simulink model "gps_navsatfix_sim"  (R2026a)
settings: Solver=FixedStepDiscrete  StopTime=Inf  FixedStep=0.1
model workspace (MAT data in the model file):
  GPS_FIX_TOPIC = '/gps/fix'
  GPS_REFERENCE_LLA = [42.3 -71.35 20]
  GPS_SAMPLE_TIME = 0.1
  ODOM_TOPIC = '/odom'
undefined symbols (not defined in the file): altitude, latitude, longitude, position_covariance, position_covariance_type, status
libraries: sensorgpslib x4, ros2lib x4
settings Model: Creator=abshanka  LastModifiedBy=abshanka
settings HardwareCC: ProdBitPerLong=64.0  ProdHWDeviceType=Intel->x86-64 (Linux 64)
settings RTWCC: SystemTargetFile=ert.tlc  HardwareBoard=Robot Operating System 2 (ROS 2)  TLCOptions="-aInlineSetEventsForThisBaseRateFcn=TLC_FALSE -aSuppressMultiTaskScheduler=TLC_FALSE  -aRateBasedStepFcn=0"  Toolchain=Colcon Tools  TargetLang=C++  Description=Embedded Coder
settings ERTTargetCC: ExtModeTransport=2.0  ExtModeAutomaticAllocSize=off  RootIOFormat=Structure reference  CodeInterfacePackaging=C++ class

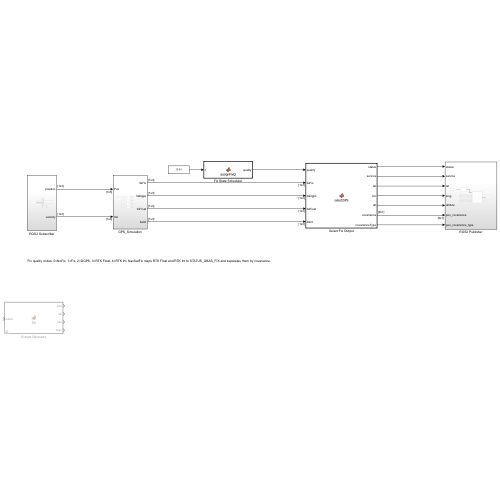
[thumbnail: Simulink's stored preview of the top-level diagram]
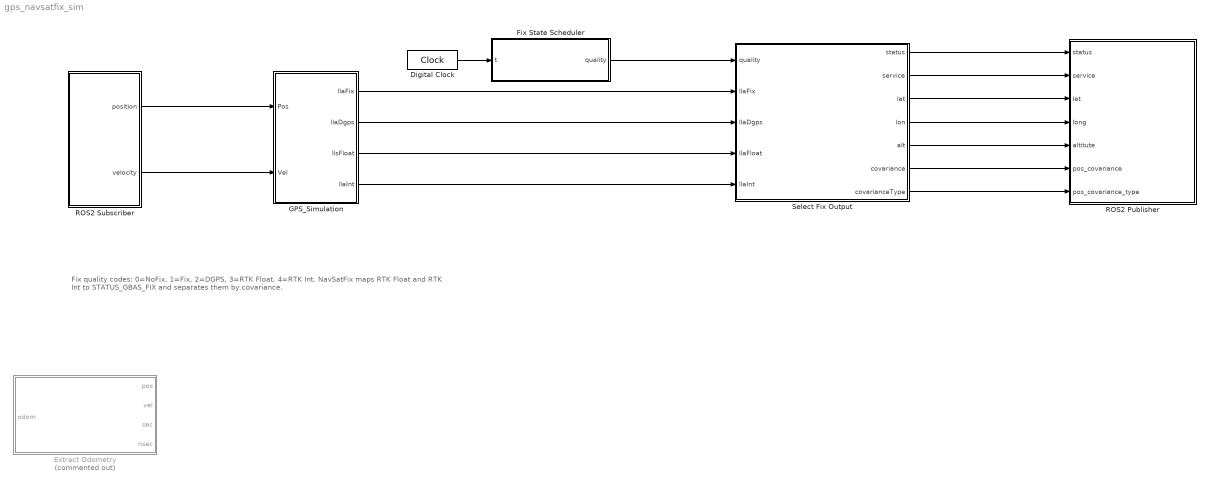
== system gps_navsatfix_sim ==
  note: Fix quality codes: 0=NoFix, 1=Fix, 2=DGPS, 3=RTK Float, 4=RTK Int. NavSatFix maps RTK Float and RTK Int to STATUS_GBAS_FIX and separates them by covariance.
  Digital Clock : DigitalClock  SampleTime=GPS_SAMPLE_TIME
  Extract Odometry : MATLAB Function  Commented=on  TreatAsAtomicUnit=on
  Fix State Scheduler : MATLAB Function  TreatAsAtomicUnit=on
  GPS_Simulation : Subsystem
  ROS2 Publisher : Subsystem
  ROS2 Subscriber : Subsystem
  Select Fix Output : MATLAB Function  TreatAsAtomicUnit=on
  wires:
  Digital Clock/1 -> Fix State Scheduler/1(t)
  Fix State Scheduler/1(quality) -> Select Fix Output/1(quality)
  GPS_Simulation/1(llaFix) -> Select Fix Output/2(llaFix)
  GPS_Simulation/2(llaDgps) -> Select Fix Output/3(llaDgps)
  GPS_Simulation/3(llsFloat) -> Select Fix Output/4(llaFloat)
  GPS_Simulation/4(llaInt) -> Select Fix Output/5(llaInt)
  ROS2 Subscriber/1(position) -> GPS_Simulation/1(Pos)
  ROS2 Subscriber/2(velocity) -> GPS_Simulation/2(Vel)
  Select Fix Output/1(status) -> ROS2 Publisher/1(status)
  Select Fix Output/2(service) -> ROS2 Publisher/2(service)
  Select Fix Output/3(lat) -> ROS2 Publisher/3(lat)
  Select Fix Output/4(lon) -> ROS2 Publisher/4(long)
  Select Fix Output/5(alt) -> ROS2 Publisher/5(altitute)
  Select Fix Output/6(covariance) -> ROS2 Publisher/6(pos_covariance)
  Select Fix Output/7(covarianceType) -> ROS2 Publisher/7(pos_covariance_type)

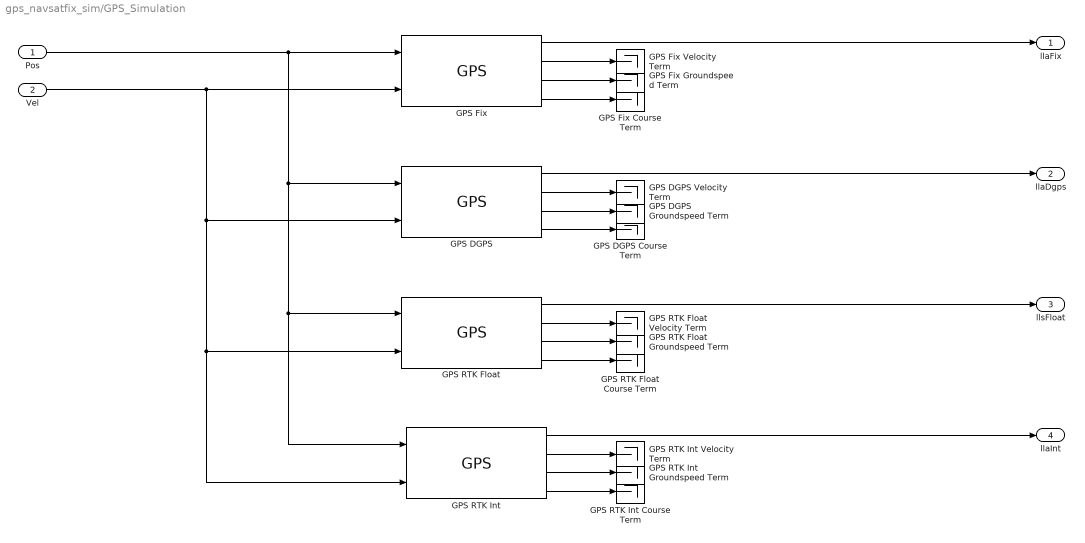
== system gps_navsatfix_sim/GPS_Simulation ==
  Pos : Inport
  Vel : Inport  Port=2
  GPS DGPS : sensorgpslib/GPS  DispRefFrame=ENU  PositionInputFormat=Local  ReferenceLocation=GPS_REFERENCE_LLA  HorizontalPositionAccuracy=0.5  VerticalPositionAccuracy=1.0  VelocityAccuracy=0.10  DecayFactor=0.999  SeedDouble=668  SimulateUsing=Interpreted execution
  GPS DGPS Course Term : Terminator
  GPS DGPS Groundspeed Term : Terminator
  GPS DGPS Velocity Term : Terminator
  GPS Fix : sensorgpslib/GPS  DispRefFrame=ENU  PositionInputFormat=Local  ReferenceLocation=GPS_REFERENCE_LLA  HorizontalPositionAccuracy=1.5  VerticalPositionAccuracy=3.0  VelocityAccuracy=0.20  DecayFactor=0.999  SeedDouble=661  SimulateUsing=Interpreted execution
  GPS Fix Course Term : Terminator
  GPS Fix Groundspeed Term : Terminator
  GPS Fix Velocity Term : Terminator
  GPS RTK Float : sensorgpslib/GPS  DispRefFrame=ENU  PositionInputFormat=Local  ReferenceLocation=GPS_REFERENCE_LLA  HorizontalPositionAccuracy=0.20  VerticalPositionAccuracy=0.40  VelocityAccuracy=0.05  DecayFactor=0.999  SeedDouble=1141  SimulateUsing=Interpreted execution
  GPS RTK Float Course Term : Terminator
  GPS RTK Float Groundspeed Term : Terminator
  GPS RTK Float Velocity Term : Terminator
  GPS RTK Int : sensorgpslib/GPS  DispRefFrame=ENU  PositionInputFormat=Local  ReferenceLocation=GPS_REFERENCE_LLA  HorizontalPositionAccuracy=0.02  VerticalPositionAccuracy=0.04  VelocityAccuracy=0.02  DecayFactor=0.999  SeedDouble=938  SimulateUsing=Interpreted execution
  GPS RTK Int Course Term : Terminator
  GPS RTK Int Groundspeed Term : Terminator
  GPS RTK Int Velocity Term : Terminator
  llaFix : Outport
  llaDgps : Outport  Port=2
  llsFloat : Outport  Port=3
  llaInt : Outport  Port=4
  wires:
  GPS Fix/2 -> GPS Fix Velocity Term/1
  GPS Fix/1 -> llaFix/1
  GPS DGPS/2 -> GPS DGPS Velocity Term/1
  GPS RTK Float/4 -> GPS RTK Float Course Term/1
  GPS RTK Float/1 -> llsFloat/1
  GPS RTK Int/4 -> GPS RTK Int Course Term/1
  GPS DGPS/3 -> GPS DGPS Groundspeed Term/1
  GPS Fix/4 -> GPS Fix Course Term/1
  GPS RTK Int/2 -> GPS RTK Int Velocity Term/1
  GPS RTK Float/2 -> GPS RTK Float Velocity Term/1
  GPS RTK Int/3 -> GPS RTK Int Groundspeed Term/1
  GPS DGPS/4 -> GPS DGPS Course Term/1
  GPS Fix/3 -> GPS Fix Groundspeed Term/1
  GPS RTK Float/3 -> GPS RTK Float Groundspeed Term/1
  GPS DGPS/1 -> llaDgps/1
  GPS RTK Int/1 -> llaInt/1
  Pos/1 -> GPS RTK Int/1, GPS RTK Float/1, GPS DGPS/1, GPS Fix/1
  Vel/1 -> GPS DGPS/2, GPS RTK Float/2, GPS RTK Int/2, GPS Fix/2

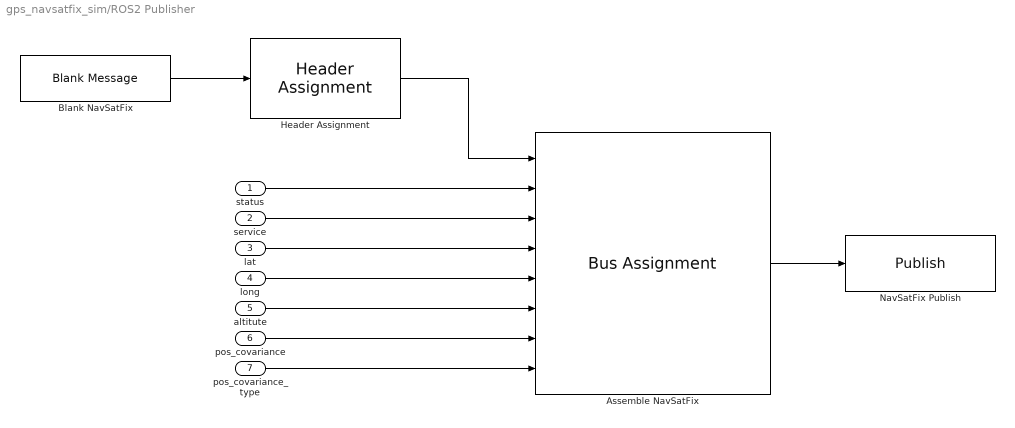
== system gps_navsatfix_sim/ROS2 Publisher ==
  status : Inport
  service : Inport  Port=2
  lat : Inport  Port=3
  long : Inport  Port=4
  altitute : Inport  Port=5
  pos_covariance : Inport  Port=6
  pos_covariance_type : Inport  Port=7
  Assemble NavSatFix : BusAssignment  AssignedSignals=status.status,status.service,latitude,longitude,altitude,position_covariance,position_covariance_type
  Blank NavSatFix : ros2lib/Blank Message  messageClass=Message  entityType=sensor_msgs/NavSatFix  messageType=sensor_msgs/NavSatFix  SampleTime=GPS_SAMPLE_TIME
  Header Assignment : ros2lib/Header Assignment  SetFrameID=off  InsertTimeStamp=on  SetHeaderFieldName=Use the default header field name  HeaderFieldName=header
  NavSatFix Publish : ros2lib/Publish  topicSource=Specify your own  topic=GPS_FIX_TOPIC  messageType=sensor_msgs/NavSatFix  QOSHistory=Keep last  QOSDepth=10  QOSReliability=Reliable  QOSDurability=Volatile  QOSDeadline=Inf  QOSLifespan=Inf  QOSLiveliness=Automatic  QOSLeaseDuration=Inf  QOSAvoidROSNamespaceConventions=off
  wires:
  pos_covariance_type/1 -> Assemble NavSatFix/8
  Assemble NavSatFix/1 -> NavSatFix Publish/1
  altitute/1 -> Assemble NavSatFix/6
  Blank NavSatFix/1 -> Header Assignment/1
  status/1 -> Assemble NavSatFix/2
  service/1 -> Assemble NavSatFix/3
  pos_covariance/1 -> Assemble NavSatFix/7
  Header Assignment/1 -> Assemble NavSatFix/1
  lat/1 -> Assemble NavSatFix/4
  long/1 -> Assemble NavSatFix/5

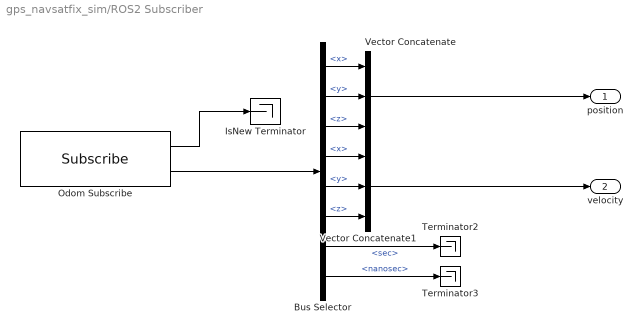
== system gps_navsatfix_sim/ROS2 Subscriber ==
  Bus Selector : BusSelector  OutputSignals=pose.pose.position.x,pose.pose.position.y,pose.pose.position.z,twist.twist.linear.x,twist.twist.linear.y,twist.twist.linear.z,header.stamp.sec,header.stamp.nanosec
  IsNew Terminator : Terminator
  Odom Subscribe : ros2lib/Subscribe  topicSource=Select from ROS network  topic=/turtle1/odom  messageType=nav_msgs/Odometry  sampleTime=GPS_SAMPLE_TIME  QOSHistory=Keep last  QOSDepth=10  QOSReliability=Reliable  QOSDurability=Volatile  QOSDeadline=Inf  QOSLifespan=Inf  QOSLiveliness=Automatic  QOSLeaseDuration=Inf  QOSAvoidROSNamespaceConventions=off
  Terminator2 : Terminator
  Terminator3 : Terminator
  Vector Concatenate : Concatenate  NumInputs=3  Mode=Multidimensional array  ConcatenateDimension=2
  Vector Concatenate1 : Concatenate  NumInputs=3  Mode=Multidimensional array  ConcatenateDimension=2
  position : Outport
  velocity : Outport  Port=2
  wires:
  Odom Subscribe/2 -> Bus Selector/1
  Bus Selector/2 -> Vector Concatenate/2  "<y>"
  Bus Selector/7 -> Terminator2/1  "<sec>"
  Bus Selector/8 -> Terminator3/1  "<nanosec>"
  Bus Selector/6 -> Vector Concatenate1/3  "<z>"
  Bus Selector/1 -> Vector Concatenate/1  "<x>"
  Odom Subscribe/1 -> IsNew Terminator/1
  Bus Selector/4 -> Vector Concatenate1/1  "<x>"
  Vector Concatenate1/1 -> velocity/1
  Bus Selector/3 -> Vector Concatenate/3  "<z>"
  Bus Selector/5 -> Vector Concatenate1/2  "<y>"
  Vector Concatenate/1 -> position/1

== matlab function gps_navsatfix_sim/Fix State Scheduler ==
  data: t input; quality output
function quality = assignFixQ(t)
%#codegen
% 0=NoFix, 1=Fix, 2=DGPS, 3=RTKFloat, 4=RTKInt
persistent nextSwitch state seed
if isempty(nextSwitch)
    nextSwitch = -1.0;
    state = uint8(4);
    seed = uint32(12345);
end
if t >= nextSwitch
    seed = uint32(mod(uint64(1664525) * uint64(seed) + uint64(1013904223), uint64(4294967296)));
    rDwell = double(seed) / 4294967295.0;
    nextSwitch = t + 5.0 + 15.0 * rDwell;
    seed = uint32(mod(uint64(1664525) * uint64(seed) + uint64(1013904223), uint64(4294967296)));
    rState = double(seed) / 4294967295.0;
    if rState < 0.45
        state = uint8(4);
    elseif rState < 0.75
        state = uint8(3);
    elseif rState < 0.85
        state = uint8(2);
    elseif rState < 0.95
        state = uint8(1);
    else
        state = uint8(0);
    end
end
quality = state;

== matlab function gps_navsatfix_sim/Extract Odometry ==
  data: odom input; pos output; vel output; sec output; nsec output
function [pos, vel, sec, nsec] = fcn(odom)
pos = [odom.pose.pose.position.x, odom.pose.pose.position.y, odom.pose.pose.position.z];
vel = [odom.twist.twist.linear.x, odom.twist.twist.linear.y, odom.twist.twist.linear.z];
sec = odom.header.stamp.sec;
nsec = odom.header.stamp.nanosec;

== matlab function gps_navsatfix_sim/Select Fix Output ==
  data: status output; service output; quality input; lat output; llaFix input; llaDgps input; llaFloat input; llaInt input; lon output; alt output; covariance output; covarianceType output
function [status, service, lat, lon, alt, covariance, covarianceType] = selectGPS(quality, llaFix, llaDgps, llaFloat, llaInt)
%#codegen
service = uint16(1);
if quality == uint8(0)
    lla = [NaN NaN NaN];
    status = int8(-1);
    hAcc = 0.0;
    vAcc = 0.0;
    covarianceType = uint8(0);
elseif quality == uint8(1)
    lla = llaFix;
    status = int8(0);
    hAcc = 1.5;
    vAcc = 3.0;
    covarianceType = uint8(2);
elseif quality == uint8(2)
    lla = llaDgps;
    status = int8(1);
    hAcc = 0.5;
    vAcc = 1.0;
    covarianceType = uint8(2);
elseif quality == uint8(3)
    lla = llaFloat;
    status = int8(2);
    hAcc = 0.20;
    vAcc = 0.40;
    covarianceType = uint8(2);
else
    lla = llaInt;
    status = int8(2);
    hAcc = 0.02;
    vAcc = 0.04;
    covarianceType = uint8(2);
end
lat = lla(1);
lon = lla(2);
alt = lla(3);
covariance = [hAcc*hAcc; 0; 0; 0; hAcc*hAcc; 0; 0; 0; vAcc*vAcc];
